simulink model "QCar_Workspace_Debug"  (R2022b)
settings: Solver=ode1  StartTime=0.0  StopTime=inf  FixedStep=1/500  RelTol=1e-3  EnableMultiTasking=on
model workspace (MAT data in the model file):
  cameraStepSize = Simulink.Parameter
  cameraStepSize.Value = Simulink.data.Expression
  cameraStepSize.Value.ExpressionString = "qc_get_step_size * 2 + 0*ceil (1/90 /qc_get_step_size)"
  cameraStepSize.DataType = 'auto'
  cameraStepSize.Complexity = 'real'
  cameraStepSize.Dimensions = -1
  internalStepSize = Simulink.Parameter
  internalStepSize.Value = Simulink.data.Expression
  internalStepSize.Value.ExpressionString = "qc_get_step_size * ceil(1/120 /qc_get_step_size)"
  internalStepSize.DataType = 'auto'
  internalStepSize.Complexity = 'real'
  internalStepSize.Dimensions = -1
  mainStepSize = Simulink.Parameter
  mainStepSize.Value = Simulink.data.Expression
  mainStepSize.Value.ExpressionString = "qc_get_step_size"
  mainStepSize.DataType = 'auto'
  mainStepSize.Complexity = 'real'
  mainStepSize.Dimensions = -1
libraries: quarc_library x30
settings Model: SimulationMode=external  ExtModeTrigDuration=10000  Creator=mbohra  LastModifiedBy=Derek
settings SolverCC: AlgebraicLoopSolver=TrustRegion  PositivePriorityOrder=on
settings DataIOCC: SaveOutput=off  SignalLogging=off  DSMLogging=off  SaveTime=off  ReturnWorkspaceOutputs=off
settings DebuggingCC: UnconnectedInputMsg=warning  UnconnectedOutputMsg=warning  UnconnectedLineMsg=warning  SFMachineParentedDataDiag=warning  ArithmeticOperatorsInVariantConditions=warning
settings ModelReferenceCC: EnableRefExpFcnMdlSchedulingChecks=on
settings SFSimCC: SimUseLocalCustomCode=off  CustomCodeUndefinedFunction=UseInterfaceOnly
settings RTWCC: Description=QUARC Win64 Target Using Toolchain  SystemTargetFile=quarc_win64.tlc  TemplateMakefile=quarc_default_tmf  RTWUseLocalCustomCode=off  Toolchain=QUARC win64 | nmake (64-bit Windows)  BuildConfiguration=Faster Runs
settings CodeAppCC: StateflowObjectComments=on
settings STFCustomTargetCC: TargetLangStandard=C99 (ISO)  ConcurrentExecutionCompliant=on  GRTInterface=on  UseToolchainInfoCompliant=on  SystemTargetFile=quarc_win64.tlc
settings GRTTargetCC: ParMdlRefBuildCompliant=off  CompOptLevelCompliant=off  CombineOutputUpdateFcns=off  MatFileLogging=off  CPPClassGenCompliant=off  GRTInterface=on  ExtMode=on  ExtModeMexFile=quarc_comm
settings ConfigComp: CovMetricSettings=dswe

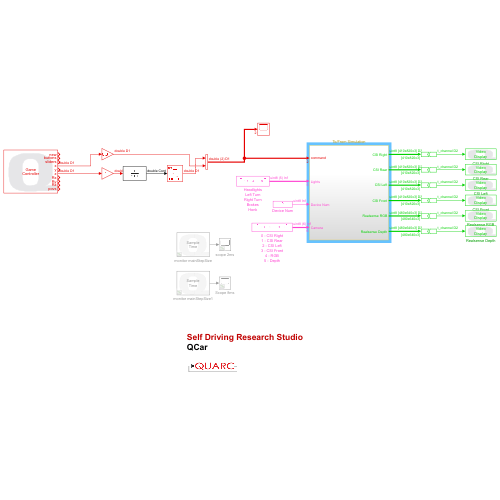
[thumbnail: Simulink's stored preview of the top-level diagram]
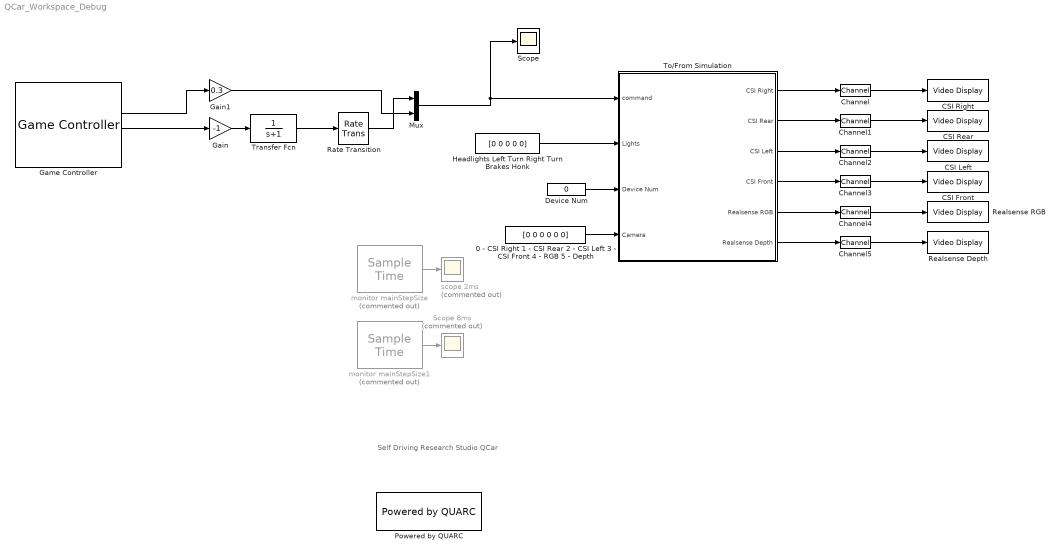
== system QCar_Workspace_Debug ==
  note: Self Driving Research Studio
      | QCar
  0 - CSI Right 1 - CSI Rear 2 - CSI Left 3 - CSI Front 4 - RGB 5 - Depth : Constant  Value=[0 0 0 0 0 0]  OutDataTypeStr=uint8
  CSI Front : quarc_library/Multimedia/Video Display  Tag=QCar_Workspace_Debug/CSI Front  sample_time=-1  use_hardware=on
  CSI Left : quarc_library/Multimedia/Video Display  Tag=QCar_Workspace_Debug/CSI Left  sample_time=-1  use_hardware=on
  CSI Rear : quarc_library/Multimedia/Video Display  Tag=QCar_Workspace_Debug/CSI Rear  sample_time=-1  use_hardware=on
  CSI Right : quarc_library/Multimedia/Video Display  Tag=QCar_Workspace_Debug/CSI Right  sample_time=-1  use_hardware=on
  Channel : quarc_library/Signal Routing/Channel  channel=0  buffer_size=1
  Channel1 : quarc_library/Signal Routing/Channel  channel=1  buffer_size=1
  Channel2 : quarc_library/Signal Routing/Channel  channel=2  buffer_size=1
  Channel3 : quarc_library/Signal Routing/Channel  channel=3  buffer_size=1
  Channel4 : quarc_library/Signal Routing/Channel  channel=4  buffer_size=1
  Channel5 : quarc_library/Signal Routing/Channel  channel=5  buffer_size=1
  Device Num : Constant  Value=0  OutDataTypeStr=uint8
  Gain : Gain  Gain=-1
  Gain1 : Gain  Gain=0.3
  Game Controller : quarc_library/Devices/Peripherals/Target/Game Controller  controller=1  buffer_size=12  deadzone=[]  saturation=[]  sample_time=qc_get_step_size  auto_center=off  enabled=on
      settings: SourceProductName=QUARC Targets
  Headlights Left Turn Right Turn Brakes Honk : Constant  Value=[0 0 0 0 0]  OutDataTypeStr=uint8
  Mux : Mux  Inputs=2
  Powered by QUARC : quarc_library/Logos/Powered by QUARC
  Rate Transition : RateTransition
  Realsense Depth : quarc_library/Multimedia/Video Display  Tag=QCar_Workspace_Debug/Realsense Depth  sample_time=-1  use_hardware=on
  Realsense RGB : quarc_library/Multimedia/Video Display  Tag=QCar_Workspace_Debug/Realsense RGB  sample_time=-1  use_hardware=on
  Scope : Scope
  Scope 8ms : Scope  Commented=on
  To/From Simulation : Subsystem
  Transfer Fcn : TransferFcn  Denominator=[1 1]
  monitor mainStepSize : quarc_library/Sources/Time/Sample Time  Priority=-99  Commented=on  sample_time=mainStepSize
  monitor mainStepSize1 : quarc_library/Sources/Time/Sample Time  Priority=-99  Commented=on  sample_time=cameraStepSize
  scope 2ms : Scope  Commented=on
  wires:
  monitor mainStepSize/1 -> scope 2ms/1
  Device Num/1 -> To/From Simulation/3(Device Num)
  Headlights Left Turn Right Turn Brakes Honk/1 -> To/From Simulation/2(Lights)
  Game Controller/4 -> Gain1/1
  Mux/1 -> Scope/1, To/From Simulation/1(command)
  Game Controller/6 -> Gain/1
  Gain/1 -> Transfer Fcn/1
  Transfer Fcn/1 -> Rate Transition/1
  Rate Transition/1 -> Mux/1
  Gain1/1 -> Mux/2
  To/From Simulation/1(CSI Right) -> Channel/1
  monitor mainStepSize1/1 -> Scope 8ms/1
  Channel/1 -> CSI Right/1
  0 - CSI Right 1 - CSI Rear 2 - CSI Left 3 - CSI Front 4 - RGB 5 - Depth/1 -> To/From Simulation/4(Camera)
  Channel1/1 -> CSI Rear/1
  To/From Simulation/2(CSI Rear) -> Channel1/1
  Channel2/1 -> CSI Left/1
  Channel3/1 -> CSI Front/1
  Channel4/1 -> Realsense RGB/1
  Channel5/1 -> Realsense Depth/1
  To/From Simulation/6(Realsense Depth) -> Channel5/1
  To/From Simulation/5(Realsense RGB) -> Channel4/1
  To/From Simulation/3(CSI Left) -> Channel2/1
  To/From Simulation/4(CSI Front) -> Channel3/1

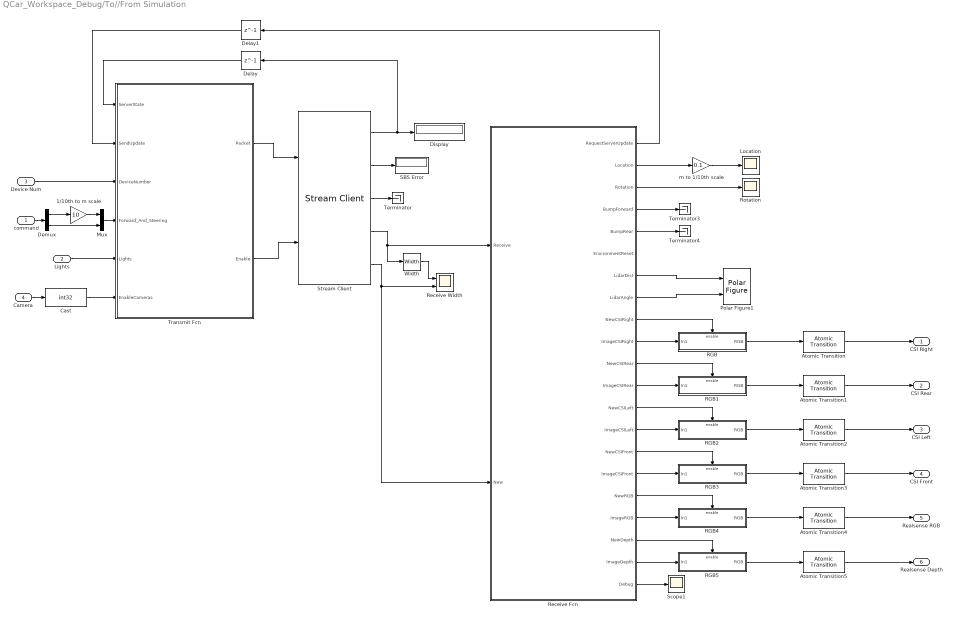
== system QCar_Workspace_Debug/To//From Simulation ==
  command : Inport
  Lights : Inport  Port=2
  Device Num : Inport  Port=3
  Camera : Inport  Port=4
  1/10th to m scale : Gain  Gain=10
  Atomic Transition{,1..5} (6 alike) : quarc_library/Advanced/Asynchronous/Atomic Transition  sample_time=0.03  data_type=Inherit: Same as input
      settings: SourceProductName=QUARC Targets
  Cast : DataTypeConversion  OutDataTypeStr=int32  SaturateOnIntegerOverflow=off  RndMeth=Floor
  Delay : Delay  DelayLength=1
  Delay1 : Delay  DelayLength=1
  Demux : Demux  Outputs=2
  Display : Display
  Location : Scope
  Mux : Mux  Inputs=2
  Polar Figure1 : quarc_library/Sinks/Figures/Polar Figure  figure_mode=Use figure window  figure_tag=figure1  axes_tag=axes1  plot_mode=Frame-based  minimum_rho=0  maximum_rho=80  minimum_theta=0  maximum_theta=360  zero_location=top  direction=clockwise  buffer_size=1  update_rate=100  sample_time=-1  initial_position="52  522  814  692"  initial_visibility=off  line1_style=None  line1_width=0.5  line1_color=[0 0.4470 0.7410]  marker1=Circle (o)  marker1_size=1  marker1_edge_color=[0 0.447059 0.741176]  marker1_face_color=[0 0.447059 0.741176]  line2_style=Solid line (-)  line2_width=0.5  line2_color=[0.85098 0.32549 0.0980392]  marker2=None  marker2_size=6  marker2_edge_color=[0.85098 0.32549 0.0980392]  marker2_face_color=[0.85098 0.32549 0.0980392]  line3_style=Solid line (-)  line3_width=0.5  line3_color=[0.929412 0.694118 0.12549]  marker3=None  marker3_size=6  marker3_edge_color=[0.929412 0.694118 0.12549]  marker3_face_color=[0.929412 0.694118 0.12549]  line4_style=Solid line (-)  line4_width=0.5  line4_color=[0.494118 0.184314 0.556863]  marker4=None  marker4_size=6  marker4_edge_color=[0.494118 0.184314 0.556863]  marker4_face_color=[0.494118 0.184314 0.556863]  line5_style=Solid line (-)  line5_width=0.5  line5_color=[0.466667 0.67451 0.188235]  marker5=None  marker5_size=6  marker5_edge_color=[0.466667 0.67451 0.188235]  marker5_face_color=[0.466667 0.67451 0.188235]
      settings: SourceProductName=QUARC Targets
  RGB : Subsystem
  RGB1 : Subsystem
  RGB2 : Subsystem
  RGB3 : Subsystem
  RGB4 : Subsystem
  RGB5 : Subsystem
  Receive Fcn : MATLAB Function  TreatAsAtomicUnit=on
  Receive Width : Scope  NumInputPorts=2
  Rotation : Scope
  SBS Error : Display
  Scope1 : Scope
  Stream Client : quarc_library/Communications/Basic/Stream Client  uri_source=Specify via dialog (do not evaluate)  uri=tcpip://localhost:18000?nagle='off'  send_buffer_size=100000  receive_buffer_size=800000  byte_order=little endian (Intel - LSB first)  optimization=Minimum latency  send_options=Send all data  receive_options=Receive all data  default_value=[0]  sample_time=qc_get_step_size  active=on  implementation=Use blocking I/O in a separate thread  send_fifo_size=2  receive_fifo_size=2  send_priority=0  receive_priority=0  send_dimensions=on  receive_dimensions=on  max_dimensions=800000  data_type=uint8  type_expr=BusObject
      settings: AttributesFormatString="\"tcpip://localhost:18000?nagle='off'\""
  Terminator : Terminator
  Terminator3 : Terminator
  Terminator4 : Terminator
  Transmit Fcn : MATLAB Function  TreatAsAtomicUnit=on
  Width : Width
  m to 1/10th scale : Gain  Gain=0.1
  CSI Right : Outport
  CSI Rear : Outport  Port=2
  CSI Left : Outport  Port=3
  CSI Front : Outport  Port=4
  Realsense RGB : Outport  Port=5
  Realsense Depth : Outport  Port=6
  wires:
  Receive Fcn/1(RequestServerUpdate) -> Delay1/1
  Stream Client/1 -> Display/1, Delay/1
  Delay1/1 -> Transmit Fcn/2(SendUpdate)
  Stream Client/3 -> Terminator/1
  Stream Client/2 -> SBS Error/1
  Stream Client/5 -> Receive Fcn/2(New), Receive Width/2
  Transmit Fcn/2(Enable) -> Stream Client/2
  Transmit Fcn/1(Packet) -> Stream Client/1
  Stream Client/4 -> Width/1, Receive Fcn/1(Receive)
  Delay/1 -> Transmit Fcn/1(ServerState)
  Device Num/1 -> Transmit Fcn/3(DeviceNumber)
  Receive Fcn/5(BumpRear) -> Terminator4/1
  Lights/1 -> Transmit Fcn/5(Lights)
  Atomic Transition/1 -> CSI Right/1
  RGB/1(RGB) -> Atomic Transition/1
  Receive Fcn/4(BumpForward) -> Terminator3/1
  Receive Fcn/3(Rotation) -> Rotation/1
  Receive Fcn/2(Location) -> m to 1/10th scale/1
  m to 1/10th scale/1 -> Location/1
  command/1 -> Demux/1
  Demux/1 -> 1/10th to m scale/1
  1/10th to m scale/1 -> Mux/1
  Demux/2 -> Mux/2
  Mux/1 -> Transmit Fcn/4(Forward_And_Steering)
  Camera/1 -> Cast/1
  Receive Fcn/7(LidarDist) -> Polar Figure1/1
  Receive Fcn/8(LidarAngle) -> Polar Figure1/2
  Receive Fcn/10(ImageCSIRight) -> RGB/1(In1)
  Receive Fcn/9(NewCSIRight) -> RGB/Enable
  Receive Fcn/21(Debug) -> Scope1/1
  Cast/1 -> Transmit Fcn/6(EnableCameras)
  Width/1 -> Receive Width/1
  Atomic Transition1/1 -> CSI Rear/1
  RGB1/1(RGB) -> Atomic Transition1/1
  Atomic Transition2/1 -> CSI Left/1
  RGB2/1(RGB) -> Atomic Transition2/1
  Atomic Transition3/1 -> CSI Front/1
  RGB3/1(RGB) -> Atomic Transition3/1
  Atomic Transition4/1 -> Realsense RGB/1
  RGB4/1(RGB) -> Atomic Transition4/1
  Atomic Transition5/1 -> Realsense Depth/1
  RGB5/1(RGB) -> Atomic Transition5/1
  Receive Fcn/20(ImageDepth) -> RGB5/1(In1)
  Receive Fcn/19(NewDepth) -> RGB5/Enable
  Receive Fcn/18(ImageRGB) -> RGB4/1(In1)
  Receive Fcn/17(NewRGB) -> RGB4/Enable
  Receive Fcn/16(ImageCSIFront) -> RGB3/1(In1)
  Receive Fcn/15(NewCSIFront) -> RGB3/Enable
  Receive Fcn/14(ImageCSILeft) -> RGB2/1(In1)
  Receive Fcn/13(NewCSILeft) -> RGB2/Enable
  Receive Fcn/12(ImageCSIRear) -> RGB1/1(In1)
  Receive Fcn/11(NewCSIRear) -> RGB1/Enable

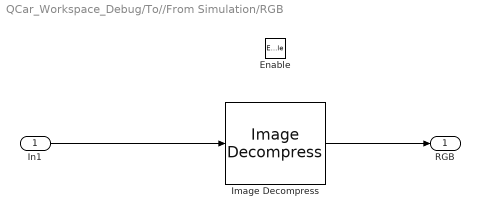
== system QCar_Workspace_Debug/To//From Simulation/RGB ==
  In1 : Inport
  Enable : EnablePort
  Image Decompress : quarc_library/Image Processing/Generic/Image Decompress  algorithm=JPEG  resolution=custom  width=820  height=410  output_format=MATLAB RGB (HxWx3)  data_type=uint8
      settings: AttributesFormatString=(%<algorithm>)  SourceProductName=QUARC Targets
  RGB : Outport  VectorParamsAs1DForOutWhenUnconnected=off
  wires:
  In1/1 -> Image Decompress/1
  Image Decompress/1 -> RGB/1

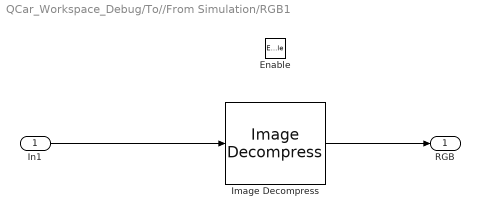
== system QCar_Workspace_Debug/To//From Simulation/RGB1 ==
  In1 : Inport
  Enable : EnablePort
  Image Decompress : quarc_library/Image Processing/Generic/Image Decompress  algorithm=JPEG  resolution=custom  width=820  height=410  output_format=MATLAB RGB (HxWx3)  data_type=uint8
      settings: AttributesFormatString=(%<algorithm>)  SourceProductName=QUARC Targets
  RGB : Outport  VectorParamsAs1DForOutWhenUnconnected=off
  wires:
  In1/1 -> Image Decompress/1
  Image Decompress/1 -> RGB/1

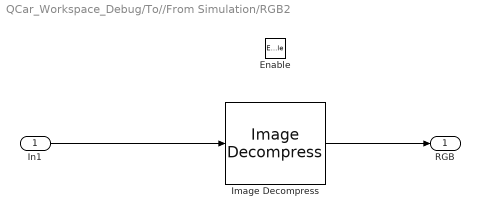
== system QCar_Workspace_Debug/To//From Simulation/RGB2 ==
  In1 : Inport
  Enable : EnablePort
  Image Decompress : quarc_library/Image Processing/Generic/Image Decompress  algorithm=JPEG  resolution=custom  width=820  height=410  output_format=MATLAB RGB (HxWx3)  data_type=uint8
      settings: AttributesFormatString=(%<algorithm>)  SourceProductName=QUARC Targets
  RGB : Outport  VectorParamsAs1DForOutWhenUnconnected=off
  wires:
  In1/1 -> Image Decompress/1
  Image Decompress/1 -> RGB/1

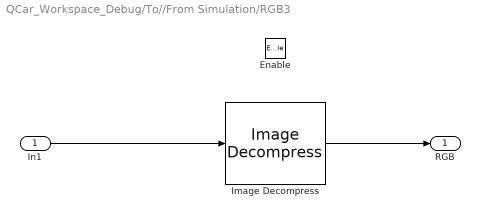
== system QCar_Workspace_Debug/To//From Simulation/RGB3 ==
  In1 : Inport
  Enable : EnablePort
  Image Decompress : quarc_library/Image Processing/Generic/Image Decompress  algorithm=JPEG  resolution=custom  width=820  height=410  output_format=MATLAB RGB (HxWx3)  data_type=uint8
      settings: AttributesFormatString=(%<algorithm>)  SourceProductName=QUARC Targets
  RGB : Outport  VectorParamsAs1DForOutWhenUnconnected=off
  wires:
  In1/1 -> Image Decompress/1
  Image Decompress/1 -> RGB/1

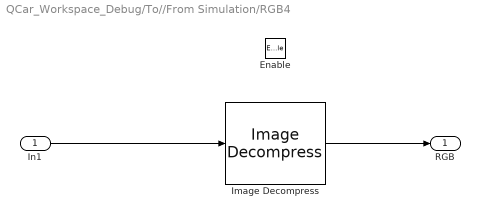
== system QCar_Workspace_Debug/To//From Simulation/RGB4 ==
  In1 : Inport
  Enable : EnablePort
  Image Decompress : quarc_library/Image Processing/Generic/Image Decompress  algorithm=JPEG  resolution=640 x 480  width=640  height=480  output_format=MATLAB RGB (HxWx3)  data_type=uint8
      settings: AttributesFormatString=(%<algorithm>)  SourceProductName=QUARC Targets
  RGB : Outport  VectorParamsAs1DForOutWhenUnconnected=off
  wires:
  In1/1 -> Image Decompress/1
  Image Decompress/1 -> RGB/1

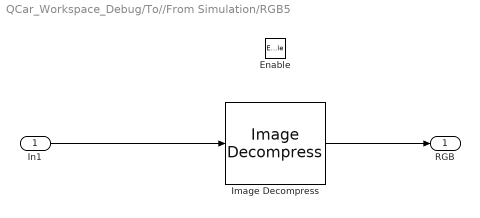
== system QCar_Workspace_Debug/To//From Simulation/RGB5 ==
  In1 : Inport
  Enable : EnablePort
  Image Decompress : quarc_library/Image Processing/Generic/Image Decompress  algorithm=JPEG  resolution=640 x 480  width=640  height=480  output_format=MATLAB RGB (HxWx3)  data_type=uint8
      settings: AttributesFormatString=(%<algorithm>)  SourceProductName=QUARC Targets
  RGB : Outport  VectorParamsAs1DForOutWhenUnconnected=off
  wires:
  In1/1 -> Image Decompress/1
  Image Decompress/1 -> RGB/1

== matlab function QCar_Workspace_Debug/To//From Simulation/Receive Fcn ==
  data: Receive input size=800000; RequestServerUpdate output; New input; Location output; Rotation output; BumpForward output; BumpRear output; EnvironmentReset output; LidarDist output; LidarAngle output; NewCSIRight output; ImageCSIRight output size=100000; NewCSIRear output; ImageCSIRear output size=100000; NewCSILeft output; ImageCSILeft output size=100000; NewCSIFront output; ImageCSIFront output size=100000; NewRGB output; ImageRGB output size=100000; NewDepth output; ImageDepth output size=100000; Debug output
function [RequestServerUpdate, Location, Rotation, BumpForward, BumpRear, EnvironmentReset, LidarDist, LidarAngle, ...
    NewCSIRight, ImageCSIRight, ...
    NewCSIRear, ImageCSIRear, ...
    NewCSILeft, ImageCSILeft, ...
    NewCSIFront, ImageCSIFront, ...
    NewRGB, ImageRGB, ...
    NewDepth, ImageDepth, ...
    Debug]  = QCarApplicationWorkspaceDecodeDataPacket(Receive, New)

%% Setup
LIDAR_SAMPLES = 384;
LIDAR_RANGE = 80;

persistent iLocation;
persistent iRotation;
persistent iBumpForward;
persistent iBumpRear;
persistent iLidarDist;
persistent iLidarAngle;

if isempty(iLocation)
    iLocation = [single(0); single(0); single(0)];
    iRotation = [single(0); single(0); single(0)];
    iBumpForward = uint8(0);
    iBumpRear = uint8(0);
    iLidarAngle = zeros(1,LIDAR_SAMPLES);   
    iLidarDist = zeros(1,LIDAR_SAMPLES);    
end

% Need to assign outputs here even though they are reassigned at the end
% since matlab can't determine the signal widths
Location = [single(0); single(0); single(0)];
Rotation = [single(0); single(0); single(0)];
BumpForward = uint8(0);
BumpRear = uint8(0);
EnvironmentReset = 0;

LidarAngle = zeros(1,LIDAR_SAMPLES);
LidarDist = zeros(1,LIDAR_SAMPLES);

ImageCSIRight = uint8([]);
NewCSIRight = 0;
ImageCSIRear = uint8([]);
NewCSIRear = 0;
ImageCSILeft = uint8([]);
NewCSILeft = 0;
ImageCSIFront = uint8([]);
NewCSIFront = 0;
ImageRGB = uint8([]);
NewRGB = 0;
ImageDepth = uint8([]);
NewDepth = 0;


RequestServerUpdate = uint8(0);
PacketSize = length(Receive);

Debug = int32(0);

% Packet > 0, new data, and magic number in first index
if ((PacketSize > 0) && (New == 1) && (Receive(1) == uint8(123)))
    
    %skip magic number
    Index = int32(2);
    
    while(Index <= PacketSize)
       
        %% Get container details
        ContainerSize = typecast(uint8(flip(Receive(Index:Index+3))), 'int32');
        DeviceID = typecast(uint8(flip(Receive(Index+4:Index+7))), 'int32');
        DeviceNum = typecast(uint8(flip(Receive(Index+8:Index+11))), 'int32');
        DeviceFunction = uint8(Receive(Index+12));
        PayloadStart = Index+13;
        PayloadEnd = Index+ContainerSize-1;
        
        %% Pass container to appropriate decoding function
        if (DeviceID == 160) %is this a QCar container?
            
            if (DeviceFunction == 11) %UE4 State Response
                [iLocation, iRotation, iBumpForward, iBumpRear] = QCarDecodeUE4VelocityStateContainer(Receive, PayloadStart);
                RequestServerUpdate = uint8(11);
            elseif (DeviceFunction == 101) % Pull out RGB payload for external processing
                CameraNum = typecast(uint8(flip(Receive(PayloadStart:PayloadStart+3))), 'int32');
                ImageSize = typecast(uint8(flip(Receive(PayloadStart+4:PayloadStart+7))), 'int32');
                
                if CameraNum == 0
                    ImageCSIRight = Receive(PayloadStart+8:PayloadEnd);
                    NewCSIRight = 1;
                    
                elseif CameraNum == 1
                    ImageCSIRear = Receive(PayloadStart+8:PayloadEnd);
                    NewCSIRear = 1;
                    
                elseif CameraNum == 2
                    ImageCSILeft = Receive(PayloadStart+8:PayloadEnd);
                    NewCSILeft = 1;
                    
                elseif CameraNum == 3
                    ImageCSIFront = Receive(PayloadStart+8:PayloadEnd);
                    NewCSIFront = 1;
                    
                elseif CameraNum == 4
                    ImageRGB = Receive(PayloadStart+8:PayloadEnd);
                    NewRGB = 1;
                    
                elseif CameraNum == 5
                    ImageDepth = Receive(PayloadStart+8:PayloadEnd);
                    NewDepth = 1;
                end
                RequestServerUpdate = uint8(1);

            elseif (DeviceFunction == 111) % Process LIDAR
                [iLidarAngle, iLidarDist] = QCarDecodeLidarContainer(Receive, PayloadStart, LIDAR_SAMPLES, LIDAR_RANGE);
                RequestServerUpdate = uint8(1);                
            end
        elseif (DeviceID == 1001) %Simulink notification
            if (DeviceFunction == 200) %Reset button
                EnvironmentReset = 1;
            end
            


        end
       
        
        %% Process next container if any data is left.
        Index = Index+ContainerSize;
    end


end

Location = iLocation;
Rotation = iRotation;
BumpForward = iBumpForward;
BumpRear = iBumpRear;
LidarDist = iLidarDist;
LidarAngle = iLidarAngle;

== matlab function QCar_Workspace_Debug/To//From Simulation/Transmit Fcn ==
  settings: updateMethod=DISCRETE  sampleTime=qc_get_step_size
  data: Packet output size=65537; ServerState input; SendUpdate input; Enable output; DeviceNumber input; Forward_And_Steering input; Lights input; EnableCameras input
function [Packet,Enable] = QCarApplicationWorkspaceMakePacketData(ServerState, SendUpdate, DeviceNumber, Forward_And_Steering, Lights, EnableCameras) 

% Be sure to set the maximum signal size of the variable size Packet port 
% in Simulink->Edit Data of the editor window.  Size should be 65537 or
% larger to ensure that the stream server generates a 4 byte packet size.

%% Setup
persistent LastServerState;

if isempty(LastServerState)
    LastServerState = uint8(0);
end

Enable = 0;
Packet = uint8([]);


%% Send new State Container or On connection
% Previous state processed, send a new one
if (SendUpdate) || ((ServerState == 2) && (LastServerState ~= 2))
    Packet = QCarMakeCommandVelocityStateContainer(DeviceNumber, Forward_And_Steering, Lights);
    
    for (index = 1:6)
        if (EnableCameras(index))
            Packet = [Packet; QCarMakeCameraRequestContainer(DeviceNumber, index-1)];
        end
    end
    Packet = [Packet; QCarMakeLidarRequestContainer(DeviceNumber)];
end

%% Transmit
% If we have data to send, enable the transmit
PacketLength = length(Packet);

if (PacketLength > 0)
    % Add magic byte.  This is just for error handling and isn't typically
    % required in simulink, but useful in lower-level languages like Python
    Packet = [uint8(123); Packet];
    
    Enable = 1; 
end


LastServerState = ServerState;
